simulink library "DoorHndDriver"  (R2022a)
settings: Solver=VariableStepAuto  StartTime=0.0  StopTime=10.0  RelTol=1e-3
settings Model: Creator=DELL  LastModifiedBy=DELL

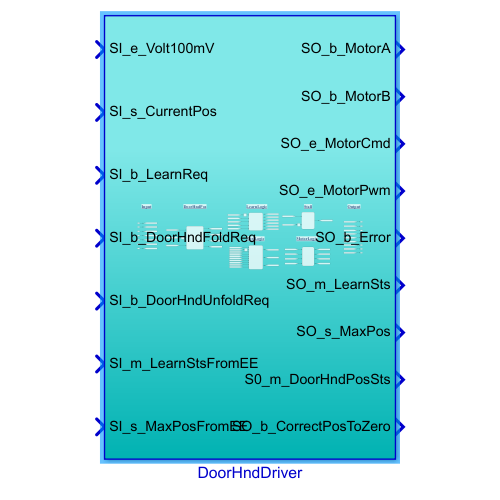
[thumbnail: Simulink's stored preview of the top-level diagram]
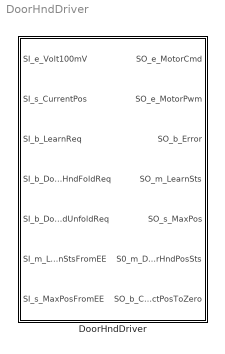
== system DoorHndDriver ==
  DoorHndDriver : Subsystem

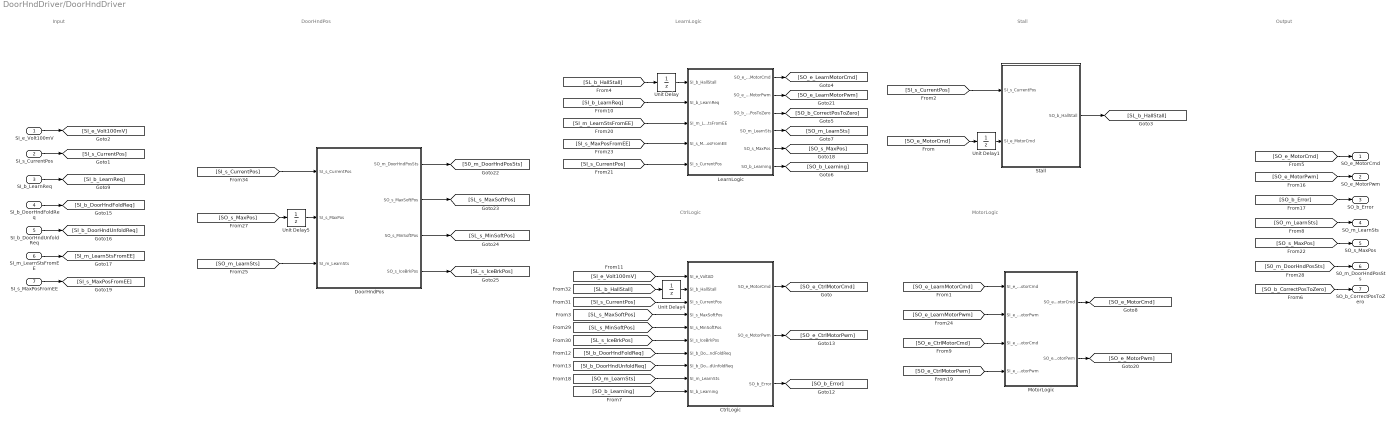
== system DoorHndDriver/DoorHndDriver ==
  note: Stall
  note: LearnLogic
  note: CtrlLogic
  note: MotorLogic
  note: Input
  note: Output
  note: DoorHndPos
  SI_e_Volt100mV : Inport
  SI_s_CurrentPos : Inport  Port=2
  SI_b_LearnReq : Inport  Port=3
  SI_b_DoorHndFoldReq : Inport  Port=4
  SI_b_DoorHndUnfoldReq : Inport  Port=5
  SI_m_LearnStsFromEE : Inport  Port=6
  SI_s_MaxPosFromEE : Inport  Port=7
  CtrlLogic : Stateflow chart  TreatAsAtomicUnit=on
  DoorHndPos : Stateflow chart  TreatAsAtomicUnit=on
  LearnLogic : Stateflow chart  TreatAsAtomicUnit=on
  MotorLogic : Stateflow chart  TreatAsAtomicUnit=on
  Stall : Stateflow chart  TreatAsAtomicUnit=on
  Unit Delay{,1,4..5} (4 alike) : UnitDelay  SampleTime=-1  HasFrameUpgradeWarning=on
  SO_e_MotorCmd : Outport
  SO_e_MotorPwm : Outport  Port=2
  SO_b_Error : Outport  Port=3
  SO_m_LearnSts : Outport  Port=4
  SO_s_MaxPos : Outport  Port=5
  S0_m_DoorHndPosSts : Outport  Port=6
  SO_b_CorrectPosToZero : Outport  Port=7
  wires:
  CtrlLogic/1(SO_e_MotorCmd) -> [SO_e_CtrlMotorCmd]
  SI_s_CurrentPos/1 -> [SI_s_CurrentPos]
  [SI_s_CurrentPos] -> Stall/1(SI_s_CurrentPos)
  SI_e_Volt100mV/1 -> [SI_e_Volt100mV]
  [SI_e_Volt100mV] -> CtrlLogic/1(SI_e_VoltAD)
  Stall/1(SO_b_HallStall) -> [SL_b_HallStall]
  [SL_b_HallStall] -> Unit Delay/1
  Unit Delay/1 -> LearnLogic/1(SI_b_HallStall)
  LearnLogic/1(SO_e_LearnMotorCmd) -> [SO_e_LearnMotorCmd]
  LearnLogic/3(SO_b_CorrectPosToZero) -> [SO_b_CorrectPosToZero]
  LearnLogic/4(SO_m_LearnSts) -> [SO_m_LearnSts]
  MotorLogic/1(SO_e_MotorCmd) -> [SO_e_MotorCmd]
  [SO_e_MotorCmd] -> Unit Delay1/1
  Unit Delay1/1 -> Stall/2(SI_e_MotorCmd)
  SI_b_LearnReq/1 -> [SI_b_LearnReq]
  [SI_b_LearnReq] -> LearnLogic/2(SI_b_LearnReq)
  CtrlLogic/3(SO_b_Error) -> [SO_b_Error]
  CtrlLogic/2(SO_e_MotorPwm) -> [SO_e_CtrlMotorPwm]
  SI_b_DoorHndFoldReq/1 -> [SI_b_DoorHndFoldReq]
  SI_b_DoorHndUnfoldReq/1 -> [SI_b_DoorHndUnfoldReq]
  [SO_e_MotorCmd] -> SO_e_MotorCmd/1
  [SO_m_LearnSts] -> SO_m_LearnSts/1
  [SO_e_MotorPwm] -> SO_e_MotorPwm/1
  [SO_b_Error] -> SO_b_Error/1
  [SI_m_LearnStsFromEE] -> LearnLogic/3(SI_m_LearnStsFromEE)
  SI_m_LearnStsFromEE/1 -> [SI_m_LearnStsFromEE]
  [SO_s_MaxPos] -> SO_s_MaxPos/1
  LearnLogic/5(SO_s_MaxPos) -> [SO_s_MaxPos]
  [SI_s_MaxPosFromEE] -> LearnLogic/4(SI_s_MaxPosFromEE)
  MotorLogic/2(SO_e_MotorPwm) -> [SO_e_MotorPwm]
  [SO_e_CtrlMotorPwm] -> MotorLogic/4(SI_e_CtrlMotorPwm)
  [SO_e_LearnMotorCmd] -> MotorLogic/1(SI_e_LearnMotorCmd)
  [SO_e_CtrlMotorCmd] -> MotorLogic/3(SI_e_CtrlMotorCmd)
  LearnLogic/2(SO_e_LearnMotorPwm) -> [SO_e_LearnMotorPwm]
  [SO_e_LearnMotorPwm] -> MotorLogic/2(SI_e_LearnMotorPwm)
  Unit Delay5/1 -> DoorHndPos/2(SI_s_MaxPos)
  DoorHndPos/1(SO_m_DoorHndPosSts) -> [S0_m_DoorHndPosSts]
  [SO_s_MaxPos] -> Unit Delay5/1
  [S0_m_DoorHndPosSts] -> S0_m_DoorHndPosSts/1
  [SO_m_LearnSts] -> CtrlLogic/9(SI_m_LearnSts)
  DoorHndPos/2(SO_s_MaxSoftPos) -> [SL_s_MaxSoftPos]
  DoorHndPos/3(SO_s_MinSoftPos) -> [SL_s_MinSoftPos]
  DoorHndPos/4(SO_s_IceBrkPos) -> [SL_s_IceBrkPos]
  [SI_s_CurrentPos] -> DoorHndPos/1(SI_s_CurrentPos)
  [SL_s_MaxSoftPos] -> CtrlLogic/4(SI_s_MaxSoftPos)
  [SL_s_MinSoftPos] -> CtrlLogic/5(SI_s_MinSoftPos)
  [SL_s_IceBrkPos] -> CtrlLogic/6(SI_s_IceBrkPos)
  [SI_b_DoorHndFoldReq] -> CtrlLogic/7(SI_b_DoorHndFoldReq)
  [SI_b_DoorHndUnfoldReq] -> CtrlLogic/8(SI_b_DoorHndUnfoldReq)
  [SI_s_CurrentPos] -> CtrlLogic/3(SI_s_CurrentPos)
  [SL_b_HallStall] -> Unit Delay4/1
  Unit Delay4/1 -> CtrlLogic/2(SI_b_HallStall)
  LearnLogic/6(SO_b_Learning) -> [SO_b_Learning]
  [SO_b_Learning] -> CtrlLogic/10(SI_b_Learning)
  SI_s_MaxPosFromEE/1 -> [SI_s_MaxPosFromEE]
  [SO_m_LearnSts] -> DoorHndPos/3(SI_m_LearnSts)
  [SI_s_CurrentPos] -> LearnLogic/5(SI_s_CurrentPos)
  [SO_b_CorrectPosToZero] -> SO_b_CorrectPosToZero/1

== stateflow chart DoorHndDriver/CtrlLogic ==
  note: SO_e_MotorCmd
      | 0: Stop A:0 B:0
      | 1: Unfold A:1 B:0
      | 2: Fold A:0 B:1
  state Ctrl
    state Idle
      en:
      SO_e_MotorCmd = 0;
      SO_e_MotorPwm = 0;
    state Unfold
      state Step2
        en:
        SO_e_MotorCmd = 1;
        SO_e_MotorPwm = 85;
      state Start
        en:
        SO_e_MotorCmd = 1;
        SO_e_MotorPwm = 100;
      state Step1
        /* 缓启 */
        en:
        SO_e_MotorCmd = 1;
        SO_e_MotorPwm = 60;
      state Icebreak
        en:
        SL_e_CycleCount = 0;
        state IceBrk
          en:
          SO_e_MotorCmd = 1;
          SO_e_MotorPwm = 100;
        state Check
          en:
          SO_e_MotorCmd = 0;
          SO_e_MotorPwm = 0;
          SL_e_CycleCount++;
        state IceBrkSuccess
          en:
          SO_e_MotorCmd = 1;
          SO_e_MotorPwm = 100;
        (default) -> IceBrk
        IceBrk -> Check : [after(50, tick)]
        Check -> IceBrk [order 3] : [after(50, tick) && ...
            | SL_e_CycleCount < 3]
        Check -> IceBrkSuccess [order 1] : [SI_s_CurrentPos > SI_s_IceBrkPos]
      state Step3
        en:
        /* 缓停 */
        SO_e_MotorCmd = 1;
        SO_e_MotorPwm = 60;
      state Stop
        en:
        SO_e_MotorCmd = 0;
        SO_e_MotorPwm = 0;
        SO_b_Error = 0;
      (default) -> (junction 617)
      Ctrl.Unfold.Step2 -> Icebreak [order 2] : [after(130, tick) && ...
          | SL_e_IceBrkCount <= 0 && ...
          | SI_s_CurrentPos < SI_s_IceBrkPos]
          | {SL_e_IceBrkCount++;}
      (junction 617) -> Ctrl.Unfold.Start [order 2] : /* 未学习 */
      (junction 617) -> Ctrl.Unfold.Step1 [order 1] : [SI_m_LearnSts == Learn_Success]
          | /* 已学习 */
      Ctrl.Unfold.Step1 -> Ctrl.Unfold.Step2 : [after(20, tick)]
      Ctrl.Unfold.Start -> Ctrl.Unfold.Stop : [after(240, tick)]
      Ctrl.Unfold.Step2 -> Ctrl.Unfold.Step3 [order 1] : [SI_s_CurrentPos >= SI_s_MaxSoftPos]
      Ctrl.Unfold.Step3 -> Ctrl.Unfold.Stop : [after(20, tick)]
      IceBrkSuccess -> Ctrl.Unfold.Step2 : [after(10, tick)]
          | {SL_e_IceBrkCount = 0;}
          | /* 破冰完成 */
    state Interrupt1
      /* 折叠打断展开 */
      en:
      SO_e_MotorCmd = 0;
      SO_e_MotorPwm = 0;
    state Interrupt2
      /* 展开打断折叠 */
      en:
      SO_e_MotorCmd = 0;
      SO_e_MotorPwm = 0;
    state Fold
      en:
      state Start
        en:
        SO_e_MotorCmd = 2;
        SO_e_MotorPwm = 100;
      state Step1
        /* 缓启 */
        en:
        SO_e_MotorCmd = 2;
        SO_e_MotorPwm = 60;
      state Step2
        en:
        SO_e_MotorCmd = 2;
        SO_e_MotorPwm = 85;
      state Step3
        en:
        /* 缓停 */
        SO_e_MotorCmd = 2;
        SO_e_MotorPwm = 60;
      state Stop
        en:
        SO_e_MotorCmd = 0;
        SO_e_MotorPwm = 0;
        SO_b_Error = 0;
      (default) -> (junction 703)
      (junction 703) -> Ctrl.Fold.Start [order 2] : /* 未学习 */
      (junction 703) -> Ctrl.Fold.Step1 [order 1] : [SI_m_LearnSts == Learn_Success]
          | /* 已学习 */
      Ctrl.Fold.Step1 -> Ctrl.Fold.Step2 : [after(20, tick)]
      Ctrl.Fold.Start -> Ctrl.Fold.Stop : [after(240, tick)]
      Ctrl.Fold.Step2 -> Ctrl.Fold.Step3 [order 1] : [SI_s_CurrentPos <= SI_s_MinSoftPos]
      Ctrl.Fold.Step3 -> Ctrl.Fold.Stop : [after(20, tick)]
    (default) -> Idle
    Ctrl.Unfold.Step2 -> Idle [order 3] : [after(200, tick)] /* 超时报错 */
    Idle -> Unfold [order 2] : [hasChangedTo(SI_b_DoorHndUnfoldReq, 1)]
    Ctrl.Unfold.Stop -> Idle
    Unfold -> Idle [order 2] : [SI_b_Learning == 1]
    Unfold -> Interrupt1 [order 1] : [hasChangedTo(SI_b_DoorHndFoldReq, 1)]
    Interrupt2 -> Unfold : after(20, tick) /* delay  */
    Interrupt1 -> Fold : after(20, tick) /* delay  */
    Fold -> Interrupt2 [order 1] : [hasChangedTo(SI_b_DoorHndUnfoldReq, 1)]
    Ctrl.Fold.Step2 -> Idle [order 2] : [after(200, tick)] /* 超时报错 */
    Idle -> Fold [order 1] : [hasChangedTo(SI_b_DoorHndFoldReq, 1)]
    Ctrl.Fold.Stop -> Idle
    Fold -> Idle [order 2] : [SI_b_Learning == 1]
    Check -> Idle [order 2] : [SL_e_CycleCount >= 3]
        | {SO_b_Error = 1;}
        | /* 破冰达到指定次数，报错 */
  data: SO_e_MotorCmd output uint8; SL_e_CycleCount local uint8; SO_e_MotorPwm output uint8; SO_b_Error output boolean; SI_e_VoltAD input uint8; SI_b_HallStall input boolean; SI_s_CurrentPos input int16; SI_s_MaxSoftPos input int16; SI_s_MinSoftPos input int16; SI_s_IceBrkPos input int16; SI_b_DoorHndFoldReq input boolean; SI_b_DoorHndUnfoldReq input boolean; SI_m_LearnSts input Enum: Learn_Sts_E; SL_e_IceBrkCount local uint8 =0; SI_b_Learning input boolean

== stateflow chart DoorHndDriver/Stall ==
  state Stall_Handler
    state Idle
      en:
      SO_b_HallStall = 0;
    state Checking
      en:
      SL_s_CurrentPos_Old = SI_s_CurrentPos;
    state Stall
      en:
      SO_b_HallStall = 1;
    Checking -> Checking [order 2] : [(SI_s_CurrentPos - SL_s_CurrentPos_Old) > 5 || ...
        | (SL_s_CurrentPos_Old - SI_s_CurrentPos) > 5]
    (default) -> Idle
    Idle -> Checking : [SI_e_MotorCmd != 0]
    Checking -> Stall [order 3] : [after(30, tick)]
    Checking -> Idle [order 1] : [SI_e_MotorCmd == 0]
    Stall -> Idle : [after(5, tick)]
  data: SL_s_CurrentPos_Old local int16; SO_b_HallStall output boolean; SI_s_CurrentPos input int16; SI_e_MotorCmd input uint8

== stateflow chart DoorHndDriver/LearnLogic ==
  state PowerOn
    en,du:
    SL_e_AutoLearnCount = 0;/*上电自动学习*/
    SO_s_MaxPos =  SI_s_MaxPosFromEE;
    SO_m_LearnSts = SI_m_LearnStsFromEE;
  note: SO_e_MotorCmd
      | 0: Stop A:0 B:0
      | 1: Unfold A:1 B:0
      | 2: Fold A:0 B:1
  state LearnLogic
    state Idle
      en:
      SO_b_Learning = 0;
      SO_e_LearnMotorCmd = 0;
      SO_e_LearnMotorPwm = 0;
      SO_b_CorrectPosToZero = 0;
    state Failed
      /* 学习失败 */
      en:
      SO_e_LearnMotorCmd = 0;
      SO_e_LearnMotorPwm = 0;
      SO_m_LearnSts = Learn_Fail;
    state Finished
      /* 学习成功 */
      en:
      SO_m_LearnSts = Learn_Success;
    state Check
      /* 学习结果判断 */
    state GotoMaxPos1
      /* 展开 */
      en,du:
      SO_b_Learning = 1;
      SO_e_LearnMotorCmd = 1;
      SO_e_LearnMotorPwm = 100;
    state Delay
      en:
      SO_e_LearnMotorCmd = 0;
      SO_e_LearnMotorPwm = 0;
    state GotoZeroPos
      /* 折叠 */
      en,du:
      SO_e_LearnMotorCmd = 2;
      SO_e_LearnMotorPwm = 100;
    state CorrectZeroPos
      /* 零点校准 */
      en:
      SO_e_LearnMotorCmd = 0;
      SO_e_LearnMotorPwm = 0;
      SO_b_CorrectPosToZero = 1;
    (default) -> Idle
    Failed -> Idle : after(3, tick)
    GotoMaxPos1 -> Failed [order 2] : [after(400, tick)]
    GotoZeroPos -> Failed [order 1] : [after(400, tick)]
    Check -> Failed [order 2]
    Check -> Finished [order 1] : [SO_s_MaxPos > 400]
    Idle -> GotoMaxPos1 [order 2] : [hasChangedTo(SI_b_LearnReq, 1)]
    CorrectZeroPos -> Check : [after(20, tick)]
    Delay -> GotoZeroPos : [after(20, tick)]
    GotoZeroPos -> CorrectZeroPos [order 2] : [SI_b_HallStall == 1]
        | {SO_s_MaxPos = (SL_e_tempPos - SI_s_CurrentPos);}
    GotoMaxPos1 -> Delay [order 1] : [SI_b_HallStall == 1]
        | {SL_e_tempPos = SI_s_CurrentPos;}
    Idle -> GotoMaxPos1 [order 1] : [SO_m_LearnSts != Learn_Success && ...
        | SL_e_AutoLearnCount > 0]
        | {SL_e_AutoLearnCount --;}
    Finished -> Idle : [after(3, tick)]
  (default) -> PowerOn
  PowerOn -> LearnLogic : [after(50, tick)] /* 500ms内读取E2学习状态和最大hall位置 */
  data: SI_b_HallStall input boolean; SO_e_LearnMotorCmd output uint8; SO_e_LearnMotorPwm output uint8; SO_b_CorrectPosToZero output boolean; SO_m_LearnSts output Enum: Learn_Sts_E; SI_b_LearnReq input boolean; SL_b_PowerOn local boolean =0; SI_m_LearnStsFromEE input Enum: Learn_Sts_E; SI_s_MaxPosFromEE input int16; SL_e_AutoLearnCount local uint8; SI_s_CurrentPos input int16; SO_s_MaxPos output int16; SL_e_tempPos local uint8; SO_b_Learning output boolean

== stateflow chart DoorHndDriver/MotorLogic ==
  state MotorLogic
    (default) -> (junction 50)
    (junction 50) -> (junction 51) [order 1] : [SI_e_LearnMotorCmd != 0]
    (junction 50) -> (junction 56) [order 2]
    (junction 51) -> (junction 59) : {SO_e_MotorCmd = SI_e_LearnMotorCmd;
        | SO_e_MotorPwm = SI_e_LearnMotorPwm;}
    (junction 56) -> (junction 61) [order 1] : [SI_e_CtrlMotorCmd != 0]
    (junction 56) -> (junction 60) [order 2] : {SO_e_MotorCmd = 0;
        | SO_e_MotorPwm = 0;}
    (junction 61) -> (junction 63) : {SO_e_MotorCmd = SI_e_CtrlMotorCmd;
        | SO_e_MotorPwm = SI_e_CtrlMotorPwm;}
    (junction 63) -> (junction 60)
    (junction 59) -> (junction 63)
    (junction 60) -> (junction 67)
  data: SO_e_MotorCmd output uint8; SO_e_MotorPwm output uint8; SI_e_LearnMotorCmd input uint8; SI_e_LearnMotorPwm input uint8; SI_e_CtrlMotorCmd input uint8; SI_e_CtrlMotorPwm input uint8

== stateflow chart DoorHndDriver/DoorHndPos ==
  state GetSoftPos
    (default) -> (junction 102)
    GetSoftPos -> (junction 102)
    (junction 102) -> (junction 103) [order 1] : [SI_m_LearnSts == Learn_Success]
    (junction 102) -> (junction 111) [order 2] : {SO_m_DoorHndPosSts = Hnd_Unknown;}
    (junction 103) -> (junction 115) : {SO_s_MaxSoftPos = SI_s_MaxPos*95/100;
        | SO_s_MinSoftPos = SI_s_MaxPos*5/100;
        | SO_s_IceBrkPos = SI_s_MaxPos*20/100;}
    (junction 115) -> (junction 242) : {SO_m_DoorHndPosSts = GetPosSts(SI_s_CurrentPos, SO_s_MinSoftPos, SO_s_MaxSoftPos);}
    (junction 242) -> (junction 111)
    (junction 111) -> (junction 117)
  state HndSts = GetPosSts(CurrentPos, MinSoftPos, MaxSoftPos) [function]
    (default) -> (junction 212)
    (junction 212) -> (junction 213) [order 1] : [CurrentPos <= MinSoftPos]
    (junction 212) -> (junction 229) [order 2]
    (junction 213) -> (junction 221) : {HndSts = Hnd_Fold;}
    (junction 229) -> (junction 219) [order 1] : [CurrentPos >=  MaxSoftPos]
    (junction 229) -> (junction 215) [order 2] : {HndSts = Hnd_Unknown;}
    (junction 219) -> (junction 226) : {HndSts = Hnd_Unfold;}
    (junction 226) -> (junction 215)
    (junction 221) -> (junction 226)
    (junction 215) -> (junction 232)
  data: CurrentPos function_input double; HndSts function_output double; MinSoftPos function_input double; MaxSoftPos function_input double; SI_s_CurrentPos input int16; SO_m_DoorHndPosSts output Enum: HndPos_Sts_E; SI_s_MaxPos input int16; SI_m_LearnSts input Enum: Learn_Sts_E; SO_s_MaxSoftPos output int16; SO_s_MinSoftPos output int16; SO_s_IceBrkPos output int16
